simulink model "scmpc"  (R2021a)
settings: Solver=VariableStepAuto  StartTime=0.0  StopTime=1859  MaxStep=0.01  RelTol=1e-3
settings Model: Creator=MQ  LastModifiedBy=MQ

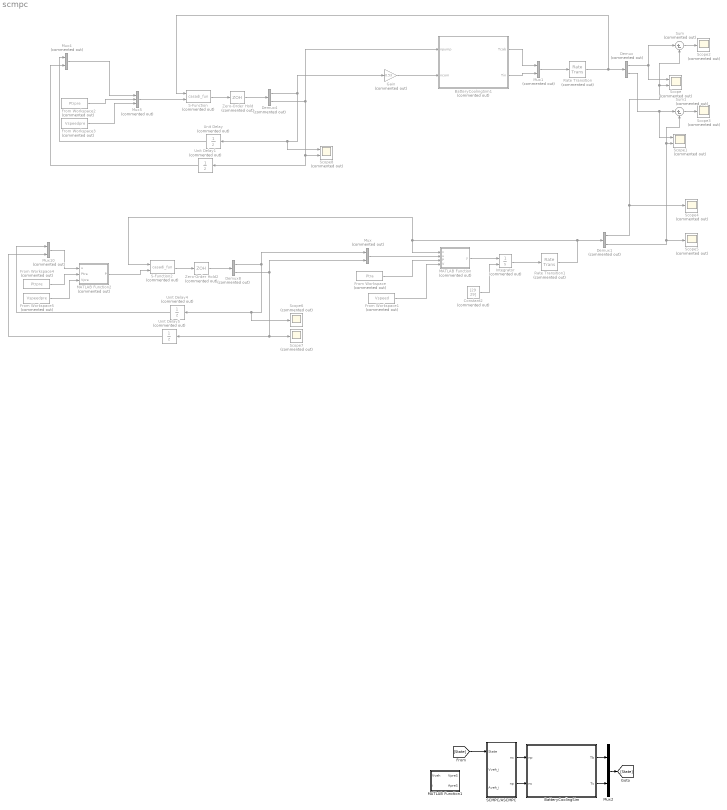
== system scmpc ==
  BatteryCoolingSim : Subsystem  Tag=AME2SL  InitFcn=AMESimLib_initBlock  StartFcn=AMESimLib_startBlock  StopFcn=AMESimLib_stopBlock
      settings: DeleteFcn=AMESimLib_deleteBlock  OpenFcn=AMESimLib_openBlock('AME2SL')
      mask Display: image(imread('amesim_pix256.png'),[0.4,0.7,0.2,0.2]);disp('Simcenter Amesim import:\nBatteryCoolingSim2');port_label('input',1,'np');port_label('input',2,'nc');port_label('output',1,'Tb');port_label('output',2,'Tc');
  BatteryCoolingSim1 : Subsystem  Tag=AME2SL  Commented=on  InitFcn=AMESimLib_initBlock  StartFcn=AMESimLib_startBlock  StopFcn=AMESimLib_stopBlock
      settings: DeleteFcn=AMESimLib_deleteBlock  OpenFcn=AMESimLib_openBlock('AME2SL')
      mask Display: image(imread('amesim_pix256.png'),[0.4,0.7,0.2,0.2]);disp('Simcenter Amesim import:\nBatteryCoolingSim');port_label('input',1,'npump');port_label('input',2,'ncom');port_label('output',1,'Tcab');port_label('output',2,'Tin');
  Constant2 : Constant  Commented=on  Value=[29 29]
  Demux{,1,4,8} (4 alike) : Demux  Commented=on  Outputs=2
  From Workspace : FromWorkspace  Commented=on  VariableName=Ptra  SampleTime=1
  From Workspace1 : FromWorkspace  Commented=on  VariableName=Vspeed  SampleTime=1
  From Workspace2 : FromWorkspace  Commented=on  VariableName=Ptrpre  SampleTime=1
  From Workspace3 : FromWorkspace  Commented=on  VariableName=Vspeedpre  SampleTime=1
  From Workspace4 : FromWorkspace  Commented=on  VariableName=Ptrpre  SampleTime=1
  From Workspace5 : FromWorkspace  Commented=on  VariableName=Vspeedpre  SampleTime=1
  Gain : Gain  Commented=on  Gain=0.53
  Integrator : Integrator  Commented=on  InitialConditionSource=external
  MATLAB Function : MATLAB Function  Commented=on  TreatAsAtomicUnit=on
  MATLAB Function1 : MATLAB Function  TreatAsAtomicUnit=on
  MATLAB Function2 : MATLAB Function  Commented=on  TreatAsAtomicUnit=on
  Mux{,1,4,10} (4 alike) : Mux  Commented=on  Inputs=2
  Mux2 : Mux  Inputs=2
  Mux5 : Mux  Commented=on  Inputs=3
  Rate Transition : RateTransition  Commented=on  InitialCondition=[29 29]  OutPortSampleTime=1
  Rate Transition1 : RateTransition  Commented=on  OutPortSampleTime=1
  S-Function : S-Function  Commented=on  FunctionName=casadi_fun  Parameters='f_mpc.casadi','f'  SFunctionDeploymentMode=off  EnableBusSupport=off
  S-Function2 : S-Function  Commented=on  FunctionName=casadi_fun  Parameters='f_scmpc.casadi','f'  SFunctionDeploymentMode=off  EnableBusSupport=off
  SCMPC/ASCMPC : Subsystem
  Scope : Scope  Commented=on  NumInputPorts=2
  Scope1 : Scope  Commented=on  NumInputPorts=2
  Scope{2..7} (6 alike) : Scope  Commented=on
  Scope8 : Scope  Commented=on  NumInputPorts=2
  Sum : Sum  Commented=on  Inputs=|+-
  Sum1 : Sum  Commented=on  Inputs=|+-
  Unit Delay{,1,4..5} (4 alike) : UnitDelay  Commented=on  InitialCondition=100  HasFrameUpgradeWarning=on
  Zero-Order Hold : ZeroOrderHold  Commented=on
  Zero-Order Hold2 : ZeroOrderHold  Commented=on
  wires:
  From Workspace/1 -> MATLAB Function/3(P)
  From Workspace1/1 -> MATLAB Function/4(V)
  Mux/1 -> MATLAB Function/2(u)
  Demux4/2 -> Unit Delay1/1, Scope8/2, BatteryCoolingSim1/1(npump)
  Demux4/1 -> Gain/1, Scope8/1, Unit Delay/1
  BatteryCoolingSim1/1(Tcab) -> Mux1/1
  Mux1/1 -> Rate Transition/1
  MATLAB Function/1(y) -> Integrator/1
  Constant2/1 -> Integrator/2
  Integrator/1 -> Rate Transition1/1
  Rate Transition/1 -> S-Function/1, Demux/1
  Demux/1 -> Sum/1, Scope/1
  Demux1/1 -> Scope4/1, Sum/2, Scope/2
  Demux/2 -> Scope1/1, Sum1/1
  Demux1/2 -> Sum1/2, Scope1/2, Scope5/1
  Sum/1 -> Scope2/1
  Sum1/1 -> Scope3/1
  S-Function/1 -> Zero-Order Hold/1
  Zero-Order Hold/1 -> Demux4/1
  Mux4/1 -> Mux5/1
  Unit Delay/1 -> Mux4/1
  Unit Delay1/1 -> Mux4/2
  Mux5/1 -> S-Function/2
  From Workspace2/1 -> Mux5/2
  From Workspace3/1 -> Mux5/3
  BatteryCoolingSim1/2(Tin) -> Mux1/2
  Gain/1 -> BatteryCoolingSim1/2(ncom)
  S-Function2/1 -> Zero-Order Hold2/1
  Demux8/1 -> Mux/1, Scope6/1, Unit Delay4/1
  Unit Delay5/1 -> Mux10/2
  Zero-Order Hold2/1 -> Demux8/1
  Rate Transition1/1 -> S-Function2/1, MATLAB Function/1(x), Demux1/1
  Unit Delay4/1 -> Mux10/1
  Demux8/2 -> Mux/2, Scope7/1, Unit Delay5/1
  Mux10/1 -> MATLAB Function2/1(u)
  From Workspace4/1 -> MATLAB Function2/2(Ptra)
  From Workspace5/1 -> MATLAB Function2/3(Vpre)
  MATLAB Function2/1(P) -> S-Function2/2
  BatteryCoolingSim/2(Tc) -> Mux2/2
  BatteryCoolingSim/1(Tb) -> Mux2/1
  SCMPC/ASCMPC/1(nc) -> BatteryCoolingSim/1(np)
  SCMPC/ASCMPC/2(np) -> BatteryCoolingSim/2(nc)
  [State] -> SCMPC/ASCMPC/1(State)
  Mux2/1 -> [State]

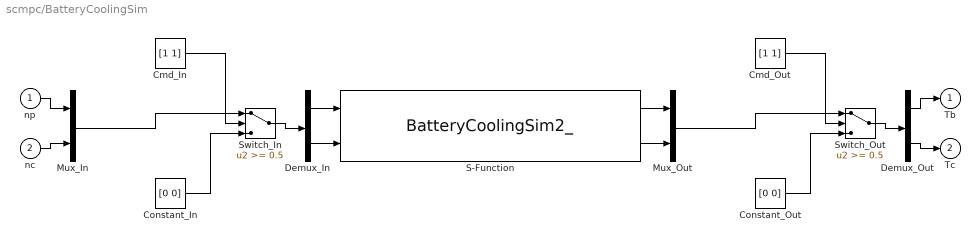
== system scmpc/BatteryCoolingSim ==
  np : Inport
  nc : Inport  Port=2
  Cmd_In : Constant  Value=[1 1]
  Cmd_Out : Constant  Value=[1 1]
  Constant_In : Constant  Value=[0 0]
  Constant_Out : Constant  Value=[0 0]
  Demux_In : Demux  Outputs=2
  Demux_Out : Demux  Outputs=2
  Mux_In : Mux  Inputs=2
  Mux_Out : Mux  Inputs=2
  S-Function : S-Function  InitFcn=clear BatteryCoolingSim_  StopFcn=clear BatteryCoolingSim_  FunctionName=BatteryCoolingSim2_  Parameters="[1,0.001] ['Gr          ';'Tamb        ';'Humidity    ';'solarFlux   ';'SOCinit     ';'Pcool       ';'posrevmax   ';'umaxfileexpr';'uminfileexpr';'Cnelem      ';'w_cell      ';'h_cell      ';'t_cell      ';'diam        ';'le          ';'condDmAirMin';'le1         ';'th_tubes    ';'pt_fins     ';'th_fins     ';'th          ';'he          ';'tamb1       ';'le_mich     ';'wi_mich     ';'he1         ';'Tinit       '] [10;30;40;700;95;1.2;12000;4.2;2.7;120;173;125;45;10;1.8;0.07065;170;2.5;1.2;0.1;35;170;30;5;1.5;170;29] ['nelems  ';'nelemp  ';'nbPipe  ';'nb_tubes';'nb_mich '] [125;2;60;10;5] [] []"  SFunctionDeploymentMode=off  EnableBusSupport=off
      mask Display: port_label('output',1,'Tcab');port_label('output',2,'Tin');port_label('input',1,'npump');port_label('input',2,'ncom');disp('Simcenter Amesim:\n BatteryCoolingSim_')
  Switch_In : Switch  Threshold=0.5  SaturateOnIntegerOverflow=on  InputSameDT=on
  Switch_Out : Switch  Threshold=0.5  SaturateOnIntegerOverflow=on  InputSameDT=on
  Tb : Outport
  Tc : Outport  Port=2
  wires:
  Mux_In/1 -> Switch_In/1
  Cmd_In/1 -> Switch_In/2
  Constant_In/1 -> Switch_In/3
  Switch_In/1 -> Demux_In/1
  Mux_Out/1 -> Switch_Out/1
  Cmd_Out/1 -> Switch_Out/2
  Constant_Out/1 -> Switch_Out/3
  Switch_Out/1 -> Demux_Out/1
  np/1 -> Mux_In/1
  Demux_In/1 -> S-Function/1
  nc/1 -> Mux_In/2
  Demux_In/2 -> S-Function/2
  Demux_Out/1 -> Tb/1
  S-Function/1 -> Mux_Out/1
  Demux_Out/2 -> Tc/1
  S-Function/2 -> Mux_Out/2

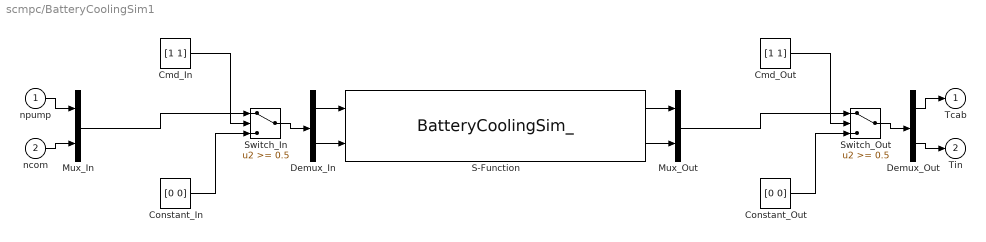
== system scmpc/BatteryCoolingSim1 ==
  npump : Inport
  ncom : Inport  Port=2
  Cmd_In : Constant  Value=[1 1]
  Cmd_Out : Constant  Value=[1 1]
  Constant_In : Constant  Value=[0 0]
  Constant_Out : Constant  Value=[0 0]
  Demux_In : Demux  Outputs=2
  Demux_Out : Demux  Outputs=2
  Mux_In : Mux  Inputs=2
  Mux_Out : Mux  Inputs=2
  S-Function : S-Function  InitFcn=clear BatteryCoolingSim_  StopFcn=clear BatteryCoolingSim_  FunctionName=BatteryCoolingSim_  Parameters="[1,0.001] ['Gr          ';'Tamb        ';'Humidity    ';'solarFlux   ';'SOCinit     ';'Pcool       ';'posrevmax   ';'umaxfileexpr';'uminfileexpr';'Cnelem      ';'w_cell      ';'h_cell      ';'t_cell      ';'diam        ';'le          ';'condDmAirMin';'le1         ';'th_tubes    ';'pt_fins     ';'th_fins     ';'th          ';'he          ';'tamb1       ';'le_mich     ';'wi_mich     ';'he1         ';'Tinit       '] [10;30;40;700;95;1.2;12000;4.2;2.7;120;173;125;45;10;1.8;0.07065;170;2.5;1.2;0.1;35;170;30;5;1.5;170;29] ['nelems  ';'nelemp  ';'nbPipe  ';'nb_tubes';'nb_mich '] [125;2;60;10;5] [] []"  SFunctionDeploymentMode=off  EnableBusSupport=off
      mask Display: port_label('output',1,'Tcab');port_label('output',2,'Tin');port_label('input',1,'npump');port_label('input',2,'ncom');disp('Simcenter Amesim:\n BatteryCoolingSim_')
  Switch_In : Switch  Threshold=0.5  SaturateOnIntegerOverflow=on  InputSameDT=on
  Switch_Out : Switch  Threshold=0.5  SaturateOnIntegerOverflow=on  InputSameDT=on
  Tcab : Outport
  Tin : Outport  Port=2
  wires:
  Mux_In/1 -> Switch_In/1
  Cmd_In/1 -> Switch_In/2
  Constant_In/1 -> Switch_In/3
  Switch_In/1 -> Demux_In/1
  Mux_Out/1 -> Switch_Out/1
  Cmd_Out/1 -> Switch_Out/2
  Constant_Out/1 -> Switch_Out/3
  Switch_Out/1 -> Demux_Out/1
  npump/1 -> Mux_In/1
  Demux_In/1 -> S-Function/1
  ncom/1 -> Mux_In/2
  Demux_In/2 -> S-Function/2
  Demux_Out/1 -> Tcab/1
  S-Function/1 -> Mux_Out/1
  Demux_Out/2 -> Tin/1
  S-Function/2 -> Mux_Out/2

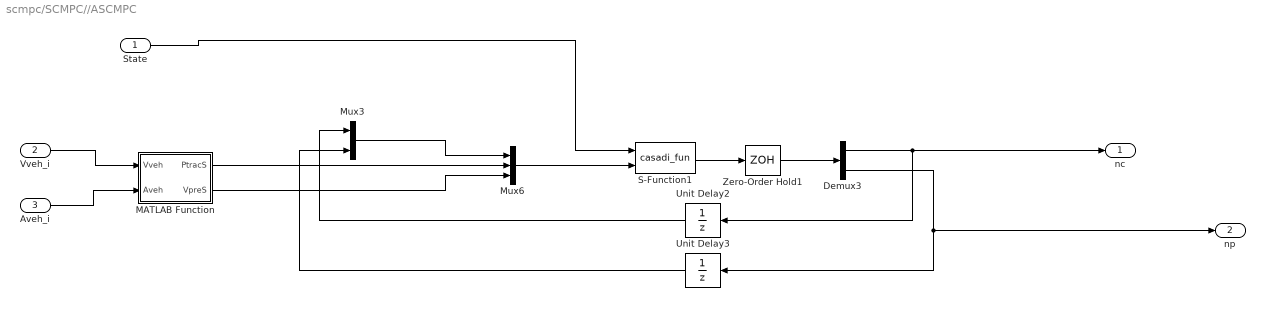
== system scmpc/SCMPC//ASCMPC ==
  State : Inport
  Vveh_i : Inport  Port=2
  Aveh_i : Inport  Port=3
  Demux3 : Demux  Outputs=2
  MATLAB Function : MATLAB Function  TreatAsAtomicUnit=on
  Mux3 : Mux  Inputs=2
  Mux6 : Mux  Inputs=3
  S-Function1 : S-Function  FunctionName=casadi_fun  Parameters='f_mpc.casadi','f'  SFunctionDeploymentMode=off  EnableBusSupport=off
  Unit Delay2 : UnitDelay  InitialCondition=100  HasFrameUpgradeWarning=on
  Unit Delay3 : UnitDelay  InitialCondition=100  HasFrameUpgradeWarning=on
  Zero-Order Hold1 : ZeroOrderHold
  nc : Outport
  np : Outport  Port=2
  wires:
  Demux3/2 -> np/1, Unit Delay3/1
  Zero-Order Hold1/1 -> Demux3/1
  Unit Delay2/1 -> Mux3/1
  Aveh_i/1 -> MATLAB Function/2(Aveh)
  Mux6/1 -> S-Function1/2
  S-Function1/1 -> Zero-Order Hold1/1
  Unit Delay3/1 -> Mux3/2
  State/1 -> S-Function1/1
  Mux3/1 -> Mux6/1
  Vveh_i/1 -> MATLAB Function/1(Vveh)
  Demux3/1 -> Unit Delay2/1, nc/1
  MATLAB Function/1(PtracS) -> Mux6/2
  MATLAB Function/2(VpreS) -> Mux6/3

== matlab function scmpc/MATLAB Function1 ==
  data: Vveh input; VpreS output; ApreS output; i input
function [VpreS,ApreS] = fcn(Vveh,i)
coder.extrinsic('evalin');
Veh=evalin('base','Veh');
Aveh=evalin('base','Aveh');
Datax=evalin('base','Datax');
S=33;

VpreS=[];
PtracS=[];
Ds=interp1(Veh(:,4),Veh(:,2),i,'pchip');  
Vt=interp1(Veh(:,4),Veh(:,1),i,'pchip');
At=Aveh(i); 
  for s=1:1:S
     Veh_hat=Datax{1,s};
     Aveh_hat=[diff(Veh_hat(:,1));0];
     [unique_x, idx] = unique(Veh_hat(:,2));unique_y = Veh_hat(idx,4);
     kk=interp1(unique_x,unique_y,Ds,'pchip');
     kk=round(kk);
     for k=1:1:N*Ts           
         hat_v=interp1(Veh_hat(:,4),Veh_hat(:,1),k+kk-1,'pchip');
         hat_Aveh=interp1(Veh_hat(:,4),Aveh_hat,k+kk-1,'pchip');
         Vse(s,k)=Vt*exp(-0.25*(k-1))+hat_v*(1-exp(-0.25*(k-1))); 
         Ase(s,k)=At*exp(-0.25*(k-1))+hat_Aveh*(1-exp(-0.25*(k-1)));
         if k+kk-1>length(Veh_hat(:,1))|Vse(s,k)>40|Vse(s,k)<0
             Vse(s,k)=0;
              Ase(s,k)=0;
         end
     end    
    [Ptrac_s, ~]=Veh_Ptrac( Vse(s,:),Ase(s,:) );
    PtracS=[PtracS,Ptrac_s(1:Ts:N*Ts)];
    VpreS=[VpreS,Vse(s,1:Ts:N*Ts)];            
  end

== matlab function scmpc/MATLAB Function ==
  data: x input; u input; y output; P input; V input
function y = rhs(x,u,P,V)
%#codegen
y =TransFun_total(x, u,P,V);

end

== matlab function scmpc/MATLAB Function2 ==
  data: u input; P output; Ptra input; Vpre input
function P = fcn(u,Ptra,Vpre)
S=8;
N=40;
p_test=zeros(2+N*2,S);
for s=1:S
    p_test(:,s)=[u(1);u(2);Ptra(1+N*(s-1):N+N*(s-1));Vpre(1+N*(s-1):N+N*(s-1))];
end
P = p_test;

== matlab function scmpc/SCMPC//ASCMPC/MATLAB Function ==
  data: Vveh input; Aveh input; PtracS output; VpreS output
function [PtracS, VpreS] = fcn(Vveh, Aveh)

[Ptrac_s, ~]=Veh_Ptrac( Vveh(:),Aveh(:) );
PtracS=[PtracS,Ptrac_s(1:Ts:N*Ts)];
VpreS=[VpreS,Vse(s,1:Ts:N*Ts)];
